simulink model "HighwayLaneChangePlanner"  (R2025b)
settings: Solver=FixedStepAuto  StartTime=0.0  StopTime=10.0  RelTol=1e-3  EnableMultiTasking=on
undefined symbols (not defined in the file): preferredLane
settings Model: Creator=The MathWorks, Inc.  LastModifiedBy=The MathWorks, Inc.
settings SolverCC: AlgebraicLoopSolver=TrustRegion  MaxZcPerStep=1.0
settings DataIOCC: SaveOutput=off
settings OptimizationCC: DefaultParameterBehavior=Inlined  InlineInvariantSignals=on  EnhancedBackFolding=on  PassReuseOutputArgsAs=Individual arguments  ZeroExternalMemoryAtStartup=off  ZeroInternalMemoryAtStartup=off  EfficientFloat2IntCast=on  OptimizeBlockOrder=speed  DifferentSizesBufferReuse=on  OptimizationCustomize=off  EfficientTunableParamExpr=on
settings DebuggingCC: ParameterTunabilityLossMsg=error  UnconnectedInputMsg=warning  UnconnectedOutputMsg=warning  UnconnectedLineMsg=warning  ModelReferenceSymbolNameMessage=none  SubsystemReferenceDiagnosticForUnitTest=warning
settings HardwareCC: ProdLongLongMode=on
settings ModelReferenceCC: EnableRefExpFcnMdlSchedulingChecks=on  ModelReferenceNumInstancesAllowed=Single  PropagateVarSize=During execution
settings RTWCC: SystemTargetFile=ert.tlc  TemplateMakefile=ert_default_tmf  RTWVerbose=off  BuildConfiguration=Faster Runs  PortableWordSizes=on  CodeExecutionProfiling=on  CodeProfilingSaveOptions=AllData  TargetLang=C++  GPUComputeCapability=3.5  DLArmComputeVersion=19.05  Description=Embedded Coder
settings CodeAppCC: ForceParamTrailComments=on  IgnoreCustomStorageClasses=off  OperatorAnnotations=on  SimulinkDataObjDesc=on  SFDataObjDesc=on  CustomSymbolStrGlobalVar=$N$M  CustomSymbolStrType=$N$M_T  CustomSymbolStrFcn=APV_$N$M$F  CustomSymbolStrMacro=$N$M  InsertBlockDesc=on
settings ERTTargetCC: RootIOFormat=Structure reference  ERTCustomFileTemplate=example_file_process.tlc  DynamicArrayContainerType=coder::array  TargetLangStandard=C++03 (ISO)  GenerateSampleERTMain=on  CombineSignalStateStructs=on  CodeInterfacePackaging=C++ class  SubcomponentCodeInterfacePackaging=C++ class  SupportVariableSizeSignals=on

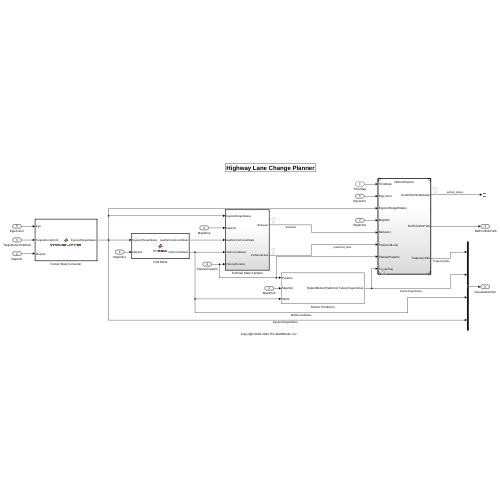
[thumbnail: Simulink's stored preview of the top-level diagram]
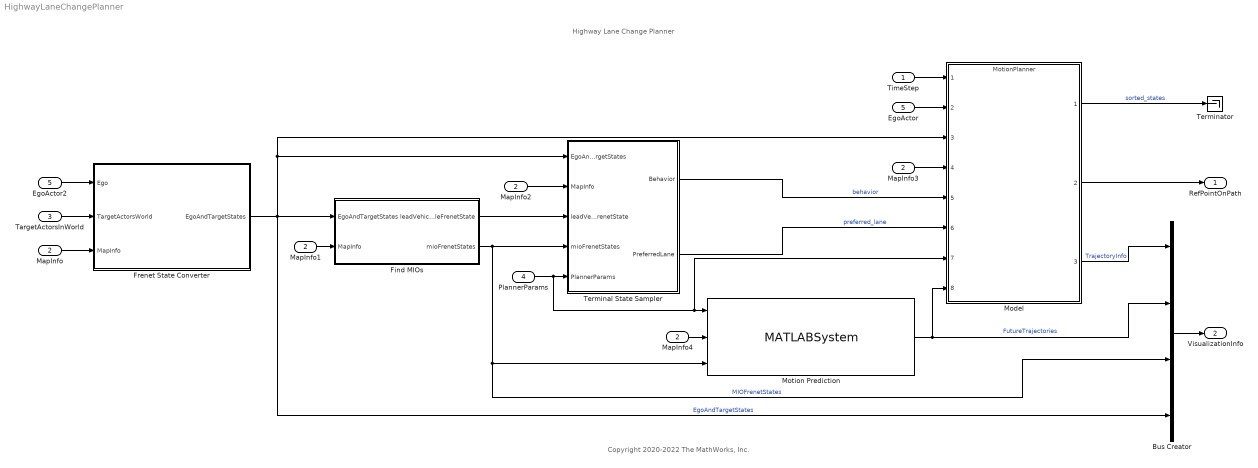
== system HighwayLaneChangePlanner ==
  note: Copyright 2020-2022 The MathWorks, Inc.
  note: Highway Lane Change Planner
  TimeStep : Inport
  MapInfo : Inport  Port=2  OutDataTypeStr=Bus: BusMapInfo  BusOutputAsStruct=on
  TargetActorsInWorld : Inport  Port=3  OutDataTypeStr=Bus: BusActorsEgo  BusOutputAsStruct=on
  PlannerParams : Inport  Port=4  OutDataTypeStr=Bus: BusPlannerParams  BusOutputAsStruct=on
  EgoActor : Inport  Port=5  OutDataTypeStr=Bus: BusVehiclePose  BusOutputAsStruct=on
  Bus Creator : BusCreator  Inputs=4
  EgoActor2 : InportShadow  Port=5  OutDataTypeStr=Bus: BusVehiclePose  BusOutputAsStruct=on
  Find MIOs : MATLAB Function  TreatAsAtomicUnit=on
  Frenet State Converter : MATLAB Function  TreatAsAtomicUnit=on
  MapInfo{1..4} (4 alike) : InportShadow  Port=2  OutDataTypeStr=Bus: BusMapInfo  BusOutputAsStruct=on
  Model : ModelReference  ModelNameDialog=MotionPlanner.slx  SimulationMode=Normal  ModelReferenceVersion=217
  Motion Prediction : MATLABSystem  System=HelperMotionPrediction  SimulateUsing=Interpreted execution
      mask Type: HelperMotionPrediction
  Terminal State Sampler : Subsystem  TreatAsAtomicUnit=on
  Terminator : Terminator
  " RefPointOnPath" : Outport  OutDataTypeStr=Bus: BusRefPointOnPath  BusOutputAsStruct=on
  VisualizationInfo : Outport  Port=2  OutDataTypeStr=Bus: BusVisualizationInfo  BusOutputAsStruct=on
  wires:
  Find MIOs/1(leadVehicleFrenetState) -> Terminal State Sampler/3(leadVehicleFrenetState)
  MapInfo3/1 -> Model/4
  EgoActor/1 -> Model/2
  Motion Prediction/1 -> Model/8, Bus Creator/2  "FutureTrajectories"
  EgoActor2/1 -> Frenet State Converter/1(Ego)
  MapInfo1/1 -> Find MIOs/2(MapInfo)
  Model/3 -> Bus Creator/1  "TrajectoryInfo"
  Frenet State Converter/1(EgoAndTargetStates) -> Bus Creator/4, Model/3, Terminal State Sampler/1(EgoAndTargetStates), Find MIOs/1(EgoAndTargetStates)  "EgoAndTargetStates"
  Terminal State Sampler/1(Behavior) -> Model/5  "behavior"
  TargetActorsInWorld/1 -> Frenet State Converter/2(TargetActorsWorld)
  MapInfo2/1 -> Terminal State Sampler/2(MapInfo)
  MapInfo/1 -> Frenet State Converter/3(MapInfo)
  TimeStep/1 -> Model/1
  Terminal State Sampler/2(PreferredLane) -> Model/6  "preferred_lane"
  MapInfo4/1 -> Motion Prediction/2
  Find MIOs/2(mioFrenetStates) -> Bus Creator/3, Motion Prediction/3, Terminal State Sampler/4(mioFrenetStates)  "MIOFrenetStates"
  Model/2 -> " RefPointOnPath"/1
  Bus Creator/1 -> VisualizationInfo/1
  PlannerParams/1 -> Model/7, Motion Prediction/1, Terminal State Sampler/5(PlannerParams)
  Model/1 -> Terminator/1  "sorted_states"

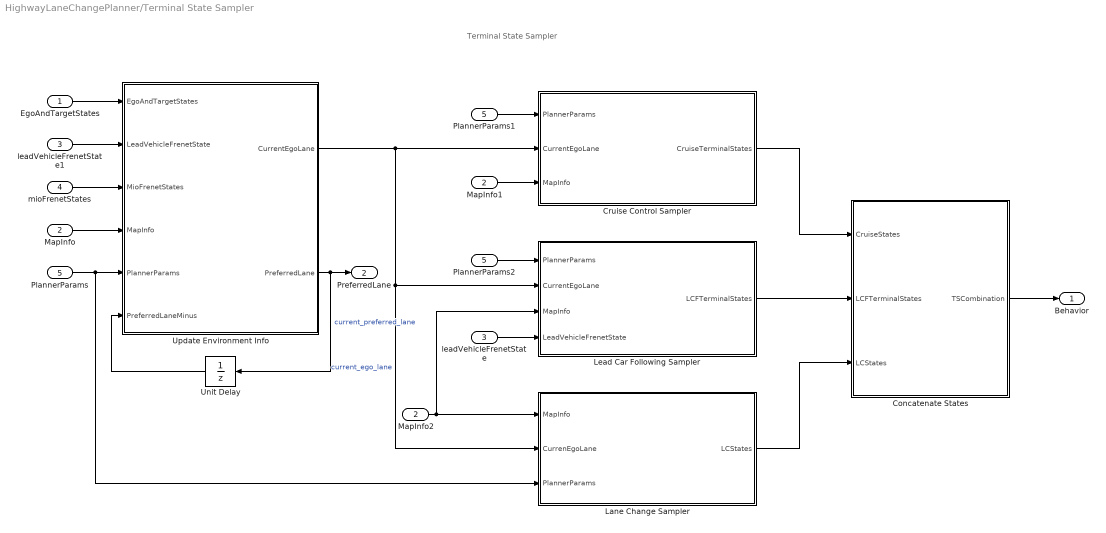
== system HighwayLaneChangePlanner/Terminal State Sampler ==
  note: Terminal State Sampler
  EgoAndTargetStates : Inport
  MapInfo : Inport  Port=2
  leadVehicleFrenetState : Inport  Port=3
  mioFrenetStates : Inport  Port=4
  PlannerParams : Inport  Port=5
  Concatenate States : MATLAB Function  TreatAsAtomicUnit=on
  Cruise Control Sampler : MATLAB Function  TreatAsAtomicUnit=on
  Lane Change Sampler : MATLAB Function  TreatAsAtomicUnit=on
  Lead Car Following Sampler : MATLAB Function  TreatAsAtomicUnit=on
  MapInfo1 : InportShadow  Port=2
  MapInfo2 : InportShadow  Port=2
  PlannerParams1 : InportShadow  Port=5
  PlannerParams2 : InportShadow  Port=5
  Unit Delay : UnitDelay  InitialCondition=preferredLane  SampleTime=-1  HasFrameUpgradeWarning=on
  Update Environment Info : MATLAB Function  TreatAsAtomicUnit=on
  leadVehicleFrenetState1 : InportShadow  Port=3
  Behavior : Outport  OutDataTypeStr=Bus: BusTerminalStatesCombinations
  PreferredLane : Outport  Port=2
  wires:
  Lane Change Sampler/1(LCStates) -> Concatenate States/3(LCStates)
  Concatenate States/1(TSCombination) -> Behavior/1
  MapInfo/1 -> Update Environment Info/4(MapInfo)
  Update Environment Info/1(CurrentEgoLane) -> Lane Change Sampler/2(CurrenEgoLane), Lead Car Following Sampler/2(CurrentEgoLane), Cruise Control Sampler/2(CurrentEgoLane)  "current_ego_lane"
  Unit Delay/1 -> Update Environment Info/6(PreferredLaneMinus)
  MapInfo2/1 -> Lane Change Sampler/1(MapInfo), Lead Car Following Sampler/3(MapInfo)
  Cruise Control Sampler/1(CruiseTerminalStates) -> Concatenate States/1(CruiseStates)
  leadVehicleFrenetState/1 -> Lead Car Following Sampler/4(LeadVehicleFrenetState)
  leadVehicleFrenetState1/1 -> Update Environment Info/2(LeadVehicleFrenetState)
  EgoAndTargetStates/1 -> Update Environment Info/1(EgoAndTargetStates)
  mioFrenetStates/1 -> Update Environment Info/3(MioFrenetStates)
  PlannerParams/1 -> Lane Change Sampler/3(PlannerParams), Update Environment Info/5(PlannerParams)
  Lead Car Following Sampler/1(LCFTerminalStates) -> Concatenate States/2(LCFTerminalStates)
  PlannerParams1/1 -> Cruise Control Sampler/1(PlannerParams)
  PlannerParams2/1 -> Lead Car Following Sampler/1(PlannerParams)
  MapInfo1/1 -> Cruise Control Sampler/3(MapInfo)
  Update Environment Info/2(PreferredLane) -> Unit Delay/1, PreferredLane/1  "current_preferred_lane"

== matlab function HighwayLaneChangePlanner/Find MIOs ==
  data: leadVehicleFrenetState output; EgoAndTargetStates input; mioFrenetStates output Bus: BusMIOFrenetStates; MapInfo input
function [leadVehicleFrenetState,...
          mioFrenetStates] =  findMIOs(EgoAndTargetStates,...
                                       MapInfo)
coder.inline('never');
%findMIOs function block identifies Most Importent Objects(MIOs) in the
%scenario.


% Get the number of target actors in the scenario from EgoAndTargetStates
% bus structure 
numTargets = EgoAndTargetStates.NumTargetActors;

% Get target actors frenet states from EgoAndTargetStates bus structure.
targetFrenetStates = EgoAndTargetStates.TargetFrenetStates;
targetIDs = EgoAndTargetStates.TargetIDs;

% Get ego actor frenet states from EgoAndTargetStates bus structure
egoFrenetState = EgoAndTargetStates.EgoFrenetState;

% Invoke the wrapper function helperFindMIOs to get the MIOs and lead
% vehicle information.
initStruct = HelperLCPlannerDefaultData.MIOFrenetStates;
mioFrenetStates = initStruct;
% Initialize lead vehicle Frenet state
leadVehicleFrenetState = inf(1,6);

% Invoke the wrapper function helperFindMIOs to get the MIOs and lead
% vehicle information.
if(numTargets)
    [mioFrenetStates,...
        leadVehicleFrenetState] =  helperFindMIOs(...,
        egoFrenetState,...
        MapInfo,...
        targetFrenetStates(1:numTargets,:),...
        targetIDs(1:numTargets,:),...
        initStruct);
end

end

== matlab function HighwayLaneChangePlanner/Frenet State Converter ==
  data: EgoAndTargetStates output Bus: BusEgoAndTargetStates; Ego input; TargetActorsWorld input; MapInfo input
function EgoAndTargetStates = frenetStateConverter(Ego,... 
                                                   TargetActorsWorld,...
                                                   MapInfo)
coder.inline('never');
persistent RefPathFrenet

refPath = MapInfo.GlobalPlanPoints(1:MapInfo.NumGlobalPlanPoints,:);
if isempty(RefPathFrenet)    
    RefPathFrenet = referencePathFrenet(refPath);   
else
    %Check for a change in the reference path
    if ~isequal(RefPathFrenet.Waypoints, refPath) 
        refPathNew = referencePathFrenet(refPath);
        RefPathFrenet.Waypoints = refPathNew.Waypoints;
    end
end

% Initialize output bus
egoAndTargetStates = HelperLCPlannerDefaultData.EgoAndTargetStates;


kapa = deg2rad(Ego.AngularVelocity(3))/norm(Ego.Velocity);
if (isnan(kapa) || isinf(kapa))
    kapa = 0;
end
egoState = [Ego.Position(1:2), deg2rad(Ego.Yaw), kapa, norm(Ego.Velocity(1:2),2), 0];%Update the acceleration state

egoFrenetState = global2frenet(RefPathFrenet, egoState);
targetStates = zeros(TargetActorsWorld.NumActors, 6);
numTargets = TargetActorsWorld.NumActors;
targetFrenetStates = zeros(numTargets, 6);
targetIDs = zeros(numTargets,1);

for i=1:numTargets
    vel = norm(TargetActorsWorld.Actors(i).Velocity(1:2));
    kappa = deg2rad(TargetActorsWorld.Actors(i).AngularVelocity(3))/vel;
    if (isnan(kappa) || isinf(kappa))
        kappa = 0;
    end

    targetStates(i,:) = [TargetActorsWorld.Actors(i).Position(1:2),...
                       deg2rad(TargetActorsWorld.Actors(i).Yaw), kappa,...
                       vel, 0];
    targetIDs(i,1) = TargetActorsWorld.Actors(i).ActorID;
    targetFrenetStates(i,:) = global2frenet(RefPathFrenet, targetStates(i,:));
    % Update the lateral and logitudinal  frenet states to zero when the
    % speed is zero.
    if abs(targetStates(i,5)) < 1e-3
        targetFrenetStates(i,2) = 0;
        targetFrenetStates(i,5) = 0;
    end
end

egoAndTargetStates.NumTargetActors = numTargets;
egoAndTargetStates.TargetGlobalStates(1:numTargets,:) = targetStates;
egoAndTargetStates.TargetFrenetStates(1:numTargets,:) = targetFrenetStates;
egoAndTargetStates.TargetIDs(1:numTargets,:) = targetIDs;
egoAndTargetStates.EgoGlobalState = egoState;
egoAndTargetStates.EgoFrenetState = egoFrenetState;
EgoAndTargetStates = egoAndTargetStates;
end

== matlab function HighwayLaneChangePlanner/Terminal State Sampler/Concatenate States ==
  data: CruiseStates input; LCFTerminalStates input; TSCombination output Bus: BusTerminalStatesCombinations; LCStates input
function TSCombination = ConcatenateStates(CruiseStates, LCFTerminalStates,...
                                           LCStates)
%ConcatenateStates concatinates the terminal states.
% The ConcatenateStates concatinates terminal states form all the behaviors
% and passes on to the down stream.

% Create and initialize terminalStateCombinations
terminalStateCombinations =  HelperLCPlannerDefaultData.TerminalStateCombinations;

%Compute valid number of states
numStates = CruiseStates.NumStates + LCStates.NumStates + LCFTerminalStates.NumStates;
terminalStateCombinations.NumCombinations = uint8(numStates);
% Update valid terminal staes into terminalStateCombinations
terminalStateCombinations.Combinations(1:numStates,1:7) = [CruiseStates.TerminalStates(1:CruiseStates.NumStates,:); LCStates.TerminalStates(1:LCStates.NumStates,:);LCFTerminalStates.TerminalStates(1:LCFTerminalStates.NumStates,:)];
for i=1:numStates
    if i <= CruiseStates.NumStates
        terminalStateCombinations.BehaviorType(i) = BehaviorType.CruiseControl;
    elseif i>CruiseStates.NumStates && i<=(LCStates.NumStates+CruiseStates.NumStates)
        terminalStateCombinations.BehaviorType(i) = BehaviorType.LaneChange;
    elseif i>(LCStates.NumStates+CruiseStates.NumStates) && i<=(LCFTerminalStates.NumStates+LCStates.NumStates+CruiseStates.NumStates)
        terminalStateCombinations.BehaviorType(i) = BehaviorType.LeadCarFollowing;
    end
end

% Assign data into output Bus veriable.
TSCombination = terminalStateCombinations;
end

== matlab function HighwayLaneChangePlanner/Terminal State Sampler/Cruise Control Sampler ==
  data: PlannerParams input; CurrentEgoLane input; MapInfo input; CruiseTerminalStates output Bus: BusTerminalStates
function CruiseTerminalStates = CruiseControlSampler(PlannerParams,...
                                                     CurrentEgoLane,...
                                                     MapInfo)
                                                     
%CruiseControlSampler samples termina states for cruise behavior.

% Create object handle for terminal state sampler class
obj = HelperTerminalStateSampler;

initStruct = HelperLCPlannerDefaultData.TerminalStates;
% Invoke cruiseControlSampler
CruiseTerminalStates = cruiseControlSampler(obj,...
                                            CurrentEgoLane,...
                                            PlannerParams.TimeHorizon,...
                                            PlannerParams.SetSpeed,...
                                            MapInfo,...
                                            PlannerParams.EnableCCBehavior,...
                                            initStruct);                                       
end

== matlab function HighwayLaneChangePlanner/Terminal State Sampler/Lane Change Sampler ==
  data: LCStates output Bus: BusTerminalStates; MapInfo input; CurrenEgoLane input; PlannerParams input
function LCStates = LaneChangeSampler(MapInfo, CurrenEgoLane,...
                                      PlannerParams)
%LaneChangeSampler samples terminal states for lane change behavior.
% The LaneChangeSampler samples termina states for lane change behavior
% using drivier setSpeed.


% Create object handle for terminal state sampler class
obj = HelperTerminalStateSampler;
initStruct = HelperLCPlannerDefaultData.TerminalStates;

% Invoke leadCarFollowingSampler
LCStates = laneChangeSampler(obj,...
                             MapInfo,...
                             CurrenEgoLane,...
                             PlannerParams,...
                             initStruct);
end

== matlab function HighwayLaneChangePlanner/Terminal State Sampler/Lead Car Following Sampler ==
  data: PlannerParams input; CurrentEgoLane input; MapInfo input; LeadVehicleFrenetState input; LCFTerminalStates output Bus: BusTerminalStates
function LCFTerminalStates = LeadCarFollowingSampler(PlannerParams,...
                                                  CurrentEgoLane,...
                                                  MapInfo,...
                                                  LeadVehicleFrenetState)
                                                     
%LeadCarFollowingSampler samples termina states for lead car following
%behavior.

% Create object handle for terminal state sampler class
obj = HelperTerminalStateSampler;
initStruct = HelperLCPlannerDefaultData.TerminalStates;

% Invoke leadCarFollowingSampler
LCFTerminalStates = leadCarFollowingSampler(obj,...
                                            CurrentEgoLane,...
                                            PlannerParams.TimeHorizon,...
                                            LeadVehicleFrenetState,...
                                            MapInfo,...
                                            PlannerParams.EnableLCFBehavior,...
                                            initStruct);
end

== matlab function HighwayLaneChangePlanner/Terminal State Sampler/Update Environment Info ==
  data: EgoAndTargetStates input; LeadVehicleFrenetState input; MioFrenetStates input; MapInfo input; PlannerParams input; PreferredLaneMinus input; CurrentEgoLane output; PreferredLane output
function [CurrentEgoLane,...
    PreferredLane] = updateEnvInfo(EgoAndTargetStates,...
    LeadVehicleFrenetState,...
    MioFrenetStates,...
    MapInfo,...
    PlannerParams,...
    PreferredLaneMinus)
%updateEnvInfo updates information about current and future lanes of ego
%along with the preferredlane.

persistent obj

% Create object handle for terminal state sampler class
if isempty(obj)
    obj = HelperTerminalStateSampler;
    obj = setUserPreferredLane(obj, PlannerParams.PreferredLane);
end

% Update ego frenet state
egoFrenetState = EgoAndTargetStates.EgoFrenetState;

% Update user preferred lane if updated
if ~isequal(obj.getUserPreferredLane(), PlannerParams.PreferredLane)    
    obj = setUserPreferredLane(obj, PlannerParams.PreferredLane);
    PreferredLaneMinus = PlannerParams.PreferredLane;    
end
initStruct = HelperLCPlannerDefaultData.MIOInfo;
% Invoke the wrapper function updateEnvironmentInfo
[CurrentEgoLane,...
 PreferredLane, ~] = updateEnvironmentInfo(obj,...
                            egoFrenetState,...
                            LeadVehicleFrenetState,...
                            MioFrenetStates,...
                            MapInfo,...
                            PlannerParams,...
                            PreferredLaneMinus,...
                            initStruct);
end
